simulink model "lin1"  (Simulink 8.1)
settings: Solver=ode45  StartTime=0.0  StopTime=10.0  RelTol=1e-3
settings Model: Creator=beard  LastModifiedBy=beard
settings DataIOCC: SignalLoggingName=sigsOut
settings OptimizationCC: InitFltsAndDblsToZero=on
settings DebuggingCC: SaveWithParameterizedLinksMsg=none  SignalResolutionControl=TryResolveAllWithWarning  SolverPrmCheckMsg=none  MultiTaskDSMMsg=warning  MultiTaskCondExecSysMsg=none  StrictBusMsg=None
settings HardwareCC: TargetUnknown=on
settings RTWCC: IncludeERTFirstTime=on

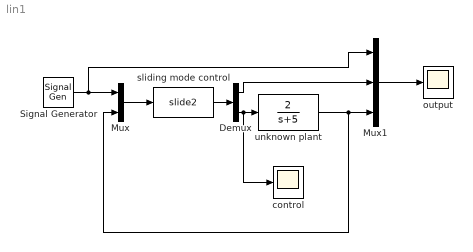
== system lin1 ==
  Demux : Demux  Outputs=2
  Mux : Mux  Inputs=2
  Mux1 : Mux  Inputs=3
  Signal Generator : SignalGenerator  WaveForm=square  Frequency=.2
  control : Scope
      settings: TimeRange=10  YMin=-3  YMax=4
  output : Scope
  sliding mode control : S-Function  FunctionName=slide2  EnableBusSupport=off
  unknown plant : TransferFcn  Numerator=[2]  Denominator=[1 5]
  wires:
  Mux/1 -> sliding mode control/1
  unknown plant/1 -> Mux/2, Mux1/3
  Signal Generator/1 -> Mux/1, Mux1/1
  Mux1/1 -> output/1
  sliding mode control/1 -> Demux/1
  Demux/2 -> unknown plant/1, control/1
  Demux/1 -> Mux1/2
